simulink model "tyreModel"  (R2013b)
settings: Solver=ode45  StartTime=0.0  StopTime=10.0  RelTol=1e-3
StartFcn:
  | tyreDataGen
values from neighbouring files (symbols this model uses):
  Rd = 0.0625    [abssim1.mat]    (also in abssim2.mat; abssim3.mat; initAbsSim.m)
  tyreData = [0 0.0585778811244 0.114421508325 0.16758915878 0.218139109665 0.266129638158 0.311619021435 0.354665536675 0.395327461053 0.433663071746 0.469730645933 0.503588460789 ... (101 elements, 1x101)]    [abssim1.mat]    (also in abssim2.mat; abssim3.mat; tyreDataGen.m = interp1(x,v,xq, 'spline'))
settings Model: Creator=kortetl1  LastModifiedBy=lasse
settings OptimizationCC: InlineParams=on
settings DebuggingCC: StateNameClashWarn=warning

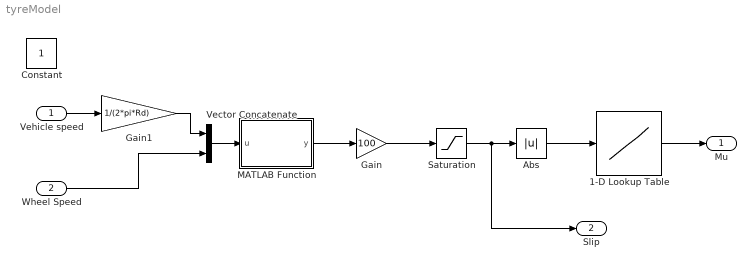
== system tyreModel ==
  Vehicle speed : Inport
  "Wheel Speed " : Inport  Port=2
  1-D Lookup Table : Lookup_n-D  NumberOfTableDimensions=1  BreakpointsForDimension1=[0:100]  Table=tyreData(1:101)  InterpMethod=Cubic spline  RndMeth=Simplest  InputSameDT=on
  Abs : Abs
  Gain : Gain  Gain=100
  Gain1 : Gain  Gain=1/(2*pi*Rd)
  MATLAB Function : MATLAB Function  TreatAsAtomicUnit=on
  Saturation : Saturate  UpperLimit=100  LowerLimit=-100
  Vector Concatenate : Concatenate
  Mu : Outport
  Slip : Outport  Port=2
  Constant : Constant  IOType=siggen
  wires:
  1-D Lookup Table/1 -> Mu/1
  Abs/1 -> 1-D Lookup Table/1
  Saturation/1 -> Slip/1, Abs/1
  Vehicle speed/1 -> Gain1/1
  "Wheel Speed "/1 -> Vector Concatenate/2
  Vector Concatenate/1 -> MATLAB Function/1(u)
  MATLAB Function/1(y) -> Gain/1
  Gain/1 -> Saturation/1
  Gain1/1 -> Vector Concatenate/1

== matlab function tyreModel/MATLAB Function ==
  data: u input; y output
function y = fcn(u)
  if u(1) == 0
      if u(2) == 0
          y = 0;
      else
          y = 1.0;
      end
  else
      if u(1) > u(2)
        y = (1 - (u(2)/u(1)))*-1;
      elseif u(2) > u(1)
        y = 1 - (u(1)/u(2));
      else
        y = 0;
      end
  end
